simulink model "acDynModel_ToLinearize_2015"  (R2015a)
settings: Solver=ode45  StartTime=0.0  StopTime=100.0  MaxStep=1e-3  RelTol=1e-3
values from neighbouring files (symbols this model uses):
  km = trim.kmass(choix)    [utGetTrimPoint.m]
  ms = trim.mStat(choix)    [utGetTrimPoint.m]
  xTrim = zeros(TOTAL_SV, 1)    [mainProjetCADV_2a.m]
undefined symbols (not defined in the file or in its folder): aircraftChosen
settings Model: CovHtmlReporting=off  Creator=thierry  LastModifiedBy=miquelth
settings DebuggingCC: UnderspecifiedInitializationDetection=Classic  MergeDetectMultiDrivingBlocksExec=none  SolverPrmCheckMsg=warning  StateNameClashWarn=warning

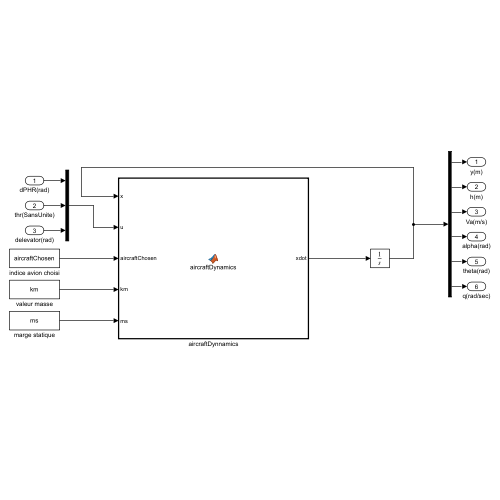
[thumbnail: Simulink's stored preview of the top-level diagram]
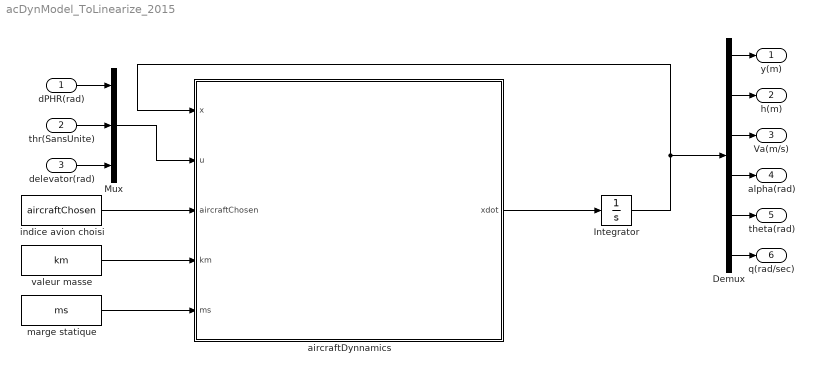
== system acDynModel_ToLinearize_2015 ==
  dPHR(rad) : Inport
  thr(SansUnite) : Inport  Port=2
  delevator(rad) : Inport  Port=3
  Demux : Demux  Outputs=6
  Integrator : Integrator  InitialCondition=xTrim
  Mux : Mux  Inputs=3
  aircraftDynnamics : MATLAB Function  TreatAsAtomicUnit=on
      settings: PermitHierarchicalResolution=ParametersOnly
  indice avion choisi : Constant  Value=aircraftChosen
  marge statique : Constant  Value=ms
  valeur masse : Constant  Value=km
  y(m) : Outport
  h(m) : Outport  Port=2
  Va(m/s) : Outport  Port=3
  alpha(rad) : Outport  Port=4
  theta(rad) : Outport  Port=5
  q(rad/sec) : Outport  Port=6
  wires:
  aircraftDynnamics/1(xdot) -> Integrator/1
  Integrator/1 -> aircraftDynnamics/1(x), Demux/1
  valeur masse/1 -> aircraftDynnamics/4(km)
  indice avion choisi/1 -> aircraftDynnamics/3(aircraftChosen)
  marge statique/1 -> aircraftDynnamics/5(ms)
  Mux/1 -> aircraftDynnamics/2(u)
  dPHR(rad)/1 -> Mux/1
  thr(SansUnite)/1 -> Mux/2
  delevator(rad)/1 -> Mux/3
  Demux/1 -> y(m)/1
  Demux/4 -> alpha(rad)/1
  Demux/5 -> theta(rad)/1
  Demux/6 -> q(rad/sec)/1
  Demux/3 -> Va(m/s)/1
  Demux/2 -> h(m)/1

== matlab function acDynModel_ToLinearize_2015/aircraftDynnamics ==
  data: x input; u input; xdot output; aircraftChosen input; km input; ms input
function xdot = aircraftDynamics(x,u, aircraftChosen,km,ms)
    TOTAL_SV = 6;
    xIn = zeros(TOTAL_SV,1);
    xIn = x;
    
	TOTAL_CMD = 3;
    uIn = zeros(TOTAL_CMD,1);
    uIn = u;
    
    xdot = utAcDynamicsFunction(xIn,uIn, aircraftChosen,km,ms);
end %aircraftDynamics
